simulink model "non_linear_vs_linear2019"  (R2019b)
settings: Solver=FixedStepAuto  StartTime=0.0  StopTime=20  FixedStep=0.001  RelTol=1e-3
values from neighbouring files (symbols this model uses):
  a = [2.10 2.14 2.2 2.3 ]    [Simulation_code.m]
  A = [730 730 730 730]    [Simulation_code.m]
  Amat = double(Amat)    [Simulation_code.m]
  Bmat = double(Bmat)    [Simulation_code.m]
  g = 981    [Simulation_code.m]
  h1_eq = 11.4    [Simulation_code.m]
  h2_eq = 11.6    [Simulation_code.m]
  h3_eq = real(double(answer.h3))    [Simulation_code.m]
  h4_eq = real(double(answer.h4))    [Simulation_code.m]
  k = [7.45 7.30]    [Simulation_code.m]
  v1_eq = real(double(answer.v1))    [Simulation_code.m]
  v2_eq = real(double(answer.v2))    [Simulation_code.m]
  y = [0.3 0.35]    [Simulation_code.m]
libraries: simulink x2
settings Model: Creator=Mostafa  LastModifiedBy=forougha
settings DebuggingCC: SFMachineParentedDataDiag=error  ArithmeticOperatorsInVariantConditions=warning
settings SFSimCC: CustomCodeUndefinedFunction=UseInterfaceOnly

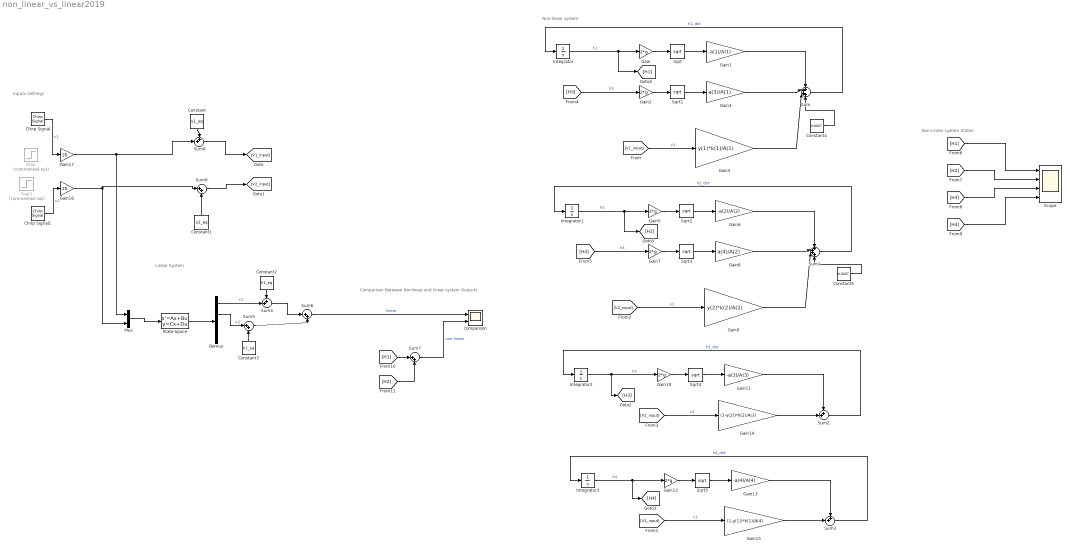
== system non_linear_vs_linear2019 ==
  note: Non-Linear syatem States
  note: Comparison Between
      | Nonlinear and linear system Outputs
  note: Non-linear system
  note: Linear System
  note: Inputs Settings
  Chirp Signal : simulink/Sources/Chirp Signal  f1=0.1  T=100  f2=1
  Chirp Signal1 : simulink/Sources/Chirp Signal  f1=0.1  T=100  f2=1
  Constant : Constant  Value=v1_eq
  Constant1 : Constant  Value=v2_eq
  Constant2 : Constant  Value=h1_eq
  Constant3 : Constant  Value=h2_eq
  Constant4 : Constant  Value=0.0037
  Constant5 : Constant  Value=0.0037
  Demux : Demux
  Gain{,2,5,7,10,12} (6 alike) : Gain  Gain=2*g
  Gain1 : Gain  Gain=-a(1)/A(1)
  Gain11 : Gain  Gain=-a(3)/A(3)
  Gain13 : Gain  Gain=-a(4)/A(4)
  Gain14 : Gain  Gain=(1-y(2))*k(2)/A(3)
  Gain15 : Gain  Gain=(1-y(1))*k(1)/A(4)
  Gain16 : Gain  Gain=20
  Gain17 : Gain  Gain=20
  Gain3 : Gain  Gain=a(3)/A(1)
  Gain4 : Gain  Gain=y(1)*k(1)/A(1)
  Gain6 : Gain  Gain=-a(2)/A(2)
  Gain8 : Gain  Gain=a(4)/A(2)
  Gain9 : Gain  Gain=y(2)*k(2)/A(2)
  Integrator : Integrator  InitialCondition=h1_eq
  Integrator1 : Integrator  InitialCondition=h2_eq
  Integrator2 : Integrator  InitialCondition=h3_eq
  Integrator3 : Integrator  InitialCondition=h4_eq
  Mux : Mux  Inputs=2
  Scope : Scope  NumInputPorts=4
  Sqrt{,1..5} (6 alike) : Sqrt  SaturateOnIntegerOverflow=on
  State-Space : StateSpace  A=Amat  B=Bmat  C=[1 0 0 0;0 1 0 0;0 0 1 0;0 0 0 1]  D=[0 0;0 0 ;0 0 ;0 0]  InitialCondition=0
  Step : Step  Commented=on  After=3.5  SampleTime=0
  Step1 : Step  Commented=on  After=3.5  SampleTime=0
  Sum : Sum  Inputs=++++
  Sum1 : Sum  Inputs=++++
  Sum{2..4,8} (4 alike) : Sum  Inputs=++|
  Sum{5..7,9} (4 alike) : Sum  Inputs=|++
  comparison : Scope  NumInputPorts=2
  wires:
  Gain/1 -> Sqrt/1
  Integrator/1 -> [H1], Gain/1  "h1"
  Sqrt/1 -> Gain1/1
  Sqrt1/1 -> Gain3/1
  [H3] -> Gain2/1  "h3"
  Gain2/1 -> Sqrt1/1
  [V1_input] -> Gain4/1  "v1"
  Gain1/1 -> Sum/1
  Gain3/1 -> Sum/2
  Gain4/1 -> Sum/3
  Sum/1 -> Integrator/1  "h1_dot"
  Sum1/1 -> Integrator1/1  "h2_dot"
  Gain9/1 -> Sum1/3
  Gain8/1 -> Sum1/2
  Gain6/1 -> Sum1/1
  [V2_input] -> Gain9/1  "v2"
  Gain7/1 -> Sqrt3/1
  [H4] -> Gain7/1  "h4"
  Sqrt3/1 -> Gain8/1
  Sqrt2/1 -> Gain6/1
  Integrator1/1 -> [H2], Gain5/1  "h2"
  Gain5/1 -> Sqrt2/1
  Gain10/1 -> Sqrt4/1
  Integrator2/1 -> [H3], Gain10/1  "h3"
  Sqrt4/1 -> Gain11/1
  [V2_input] -> Gain14/1  "v2"
  Gain11/1 -> Sum2/1
  Sum2/1 -> Integrator2/1  "h3_dot"
  Gain14/1 -> Sum2/2
  Gain15/1 -> Sum3/2
  Sum3/1 -> Integrator3/1  "h4_dot"
  Gain13/1 -> Sum3/1
  [V1_input] -> Gain15/1  "v1"
  Sqrt5/1 -> Gain13/1
  Integrator3/1 -> [H4], Gain12/1  "h4"
  Gain12/1 -> Sqrt5/1
  [H1] -> Scope/1
  [H2] -> Scope/2
  [H3] -> Scope/3
  [H4] -> Scope/4
  Mux/1 -> State-Space/1
  State-Space/1 -> Demux/1
  Demux/1 -> Sum4/2  "x1"
  Demux/2 -> Sum5/1  "x2"
  Constant2/1 -> Sum4/1
  Constant3/1 -> Sum5/2
  Sum4/1 -> Sum6/1
  Sum5/1 -> Sum6/2
  Sum6/1 -> comparison/1  "linear"
  [H1] -> Sum7/1
  [H2] -> Sum7/2
  Sum7/1 -> comparison/2  "non-linear"
  Constant/1 -> Sum8/1
  Sum8/1 -> [V1_input]
  Constant1/1 -> Sum9/2
  Sum9/1 -> [V2_input]
  Gain16/1 -> Sum9/1, Mux/2
  Gain17/1 -> Mux/1, Sum8/2
  Constant4/1 -> Sum/4
  Constant5/1 -> Sum1/4
  Chirp Signal1/1 -> Gain16/1  "v2"
  Chirp Signal/1 -> Gain17/1  "v1"
